simulink model "faultdetectsimulink2"  (R2024b)
settings: Solver=VariableStepAuto  StartTime=0.0  StopTime=0.05  RelTol=1e-3
undefined symbols (not defined in the file or in its folder): D1, Delta
libraries: spsCurrentMeasurementLib x4, spsDistributedParametersLineLib x2, spsThreePhaseVIMeasurementLib x2, spsThreePhaseParallelRLCLoadLib x1, spsThreePhaseTransformerTwoWindingsLib x1, spsThreePhaseFaultLib x1, spsThreePhaseSourceLib x1, sps_lib x1

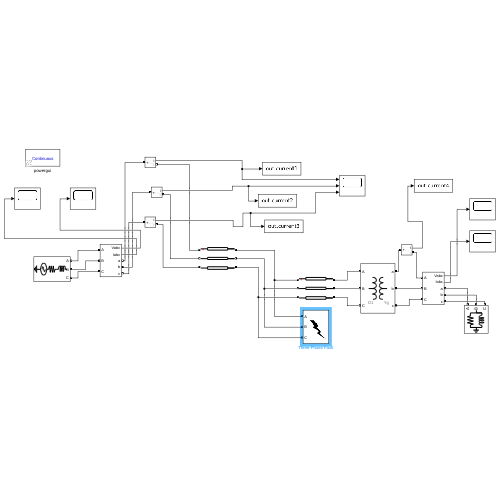
[thumbnail: Simulink's stored preview of the top-level diagram]
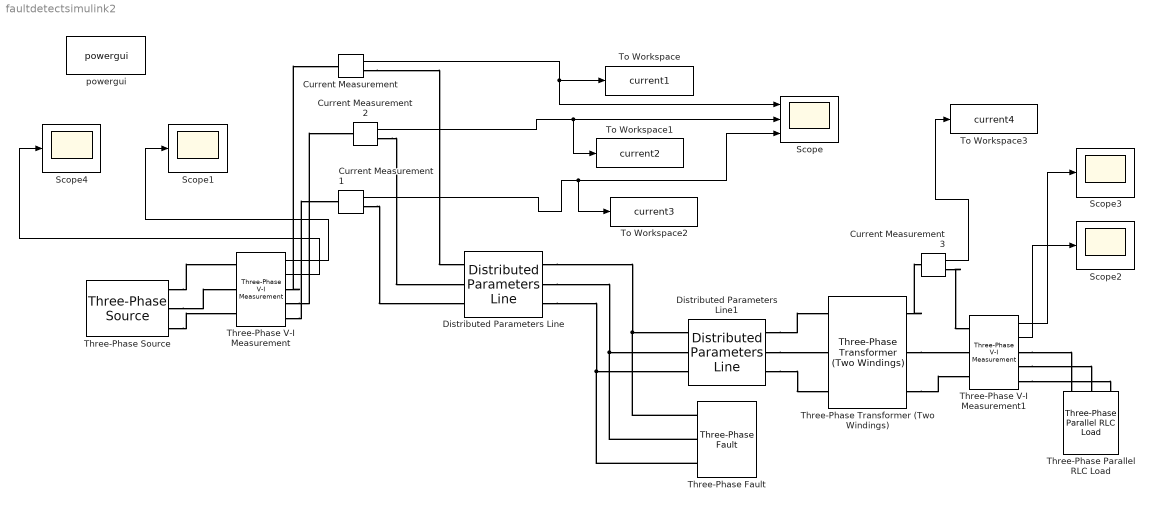
== system faultdetectsimulink2 ==
  Current Measurement{,1..3} (4 alike) : spsCurrentMeasurementLib/Current Measurement  PhasorSimulation=off  OutputType=Complex  PSBequivalent=0
  Distributed Parameters Line : spsDistributedParametersLineLib/Distributed Parameters Line  Phases=3  Length=50  Frequency=50  Resistance=[0.01273 0.3864]  Inductance="[0.9337e-3  4.1264e-3]"  Capacitance=[12.74e-9 7.751e-9]  x1=[3.31061068631267e-12 10912.2714652034 10912.2714652034;314.159265358979 314.159265358979 314.159265358979;-0.367134720613786 0.462312277142197 -1.1084840496527]  x2=[2.03369197834017e-12 10685.5908410511 10685.5908410511;314.159265358979 314.159265358979 314.159265358979;2.58910998298031 0.439349659693703 -1.13144666710119]  x3=[7.88847070447316e-14 26.7116749403581 26.7116749403585;314.159265358979 314.159265358979 314.159265358979;1.48196126518622 1.00491715671543 -0.565879170079457]  x4=[8.43670802456055e-14 59.1805317893528 59.1805317893527;314.159265358979 314.159265358979 314.159265358979;-1.58684353979965 0.173480669902326 -1.39731565689257]  x5=0.000282770783497871  V1=[3.311e-12 1.091e+04 1.091e+04;314.2 314.2 314.2;-0.3671 0.4623 -1.108]  V2=[2.034e-12 1.069e+04 1.069e+04;314.2 314.2 314.2;2.589 0.4393 -1.131]  I1=[7.888e-14 26.71 26.71;314.2 314.2 314.2;1.482 1.005 -0.5659]  I2=[8.437e-14 59.18 59.18;314.2 314.2 314.2;-1.587 0.1735 -1.397]  nHarmo=1  Measurements=None  Decoupling=off  VsMag0=0  VrMag0=0  VsAngle0=0  VrAngle0=0  IsMag0=0  IrMag0=0  IsAngle0=0  IrAngle0=0
      settings: LibrarySourceBlock=sps_lib/Power Grid Elements/Distributed Parameters Line
  Distributed Parameters Line1 : spsDistributedParametersLineLib/Distributed Parameters Line  Phases=3  Length=50  Frequency=50  Resistance=[0.01273 0.3864]  Inductance="[0.9337e-3  4.1264e-3]"  Capacitance=[12.74e-9 7.751e-9]  x1=[2.03369197834017e-12 10685.5908410511 10685.5908410511;314.159265358979 314.159265358979 314.159265358979;2.58910998298031 0.439349659693703 -1.13144666710119]  x2=[1.03798012883211e-11 10433.4111825919 10433.4111825918;314.159265358979 314.159265358979 314.159265358979;-2.16247459933143 0.415478379478156 -1.15531794731674]  x3=[2.26197302864717e-13 26.7063441276431 26.7063441276433;314.159265358979 314.159265358979 314.159265358979;3.02950596917066 1.06083330674248 -0.509963020052391]  x4=[1.49037955982956e-13 59.1198595873729 59.1198595873732;314.159265358979 314.159265358979 314.159265358979;0.100486855906676 0.119677432982979 -1.45111889381193]  x5=0.000282770783497871  V1=[2.034e-12 1.069e+04 1.069e+04;314.2 314.2 314.2;2.589 0.4393 -1.131]  V2=[1.038e-11 1.043e+04 1.043e+04;314.2 314.2 314.2;-2.162 0.4155 -1.155]  I1=[2.262e-13 26.71 26.71;314.2 314.2 314.2;3.03 1.061 -0.51]  I2=[1.49e-13 59.12 59.12;314.2 314.2 314.2;0.1005 0.1197 -1.451]  nHarmo=1  Measurements=None  Decoupling=off  VsMag0=0  VrMag0=0  VsAngle0=0  VrAngle0=0  IsMag0=0  IrMag0=0  IsAngle0=0  IrAngle0=0
      settings: LibrarySourceBlock=sps_lib/Power Grid Elements/Distributed Parameters Line
  Scope : Scope  NumInputPorts=3
  Scope{1..4} (4 alike) : Scope
  Three-Phase Parallel RLC Load : spsThreePhaseParallelRLCLoadLib/Three-Phase Parallel RLC Load  LConnTagsString=A|B|C  Configuration=Y (grounded)  NominalVoltage=400  Vabc=[1e3 1e3 1e3]  Vabcp=[1e3 1e3 1e3]  NominalFrequency=50  UnbalancedPower=off  ActivePower=10e3  InductivePower=100  CapacitivePower=0  Pabc=[10e3 9e3 11e3]  QLabc=[100 90 110]  QCabc=[100 90 110]  Pabcp=[10e3 9e3 11e3]  QLabcp=[100 90 110]  QCabcp=[100 90 110]  Measurements=None  LoadType=constant Z
  Three-Phase Transformer (Two Windings) : spsThreePhaseTransformerTwoWindingsLib/Three-Phase Transformer (Two Windings)  Winding1Connection=Delta (D1)  Winding2Connection=Yg  CoreType=Three single-phase transformers  SetSaturation=off  Hysteresis=off  DataFile='hysteresis'  SetInitialFlux=off  Measurements=None  UNITS=pu  NominalPower=[ 100e6 , 50 ]  Winding1=[ 11e3 , 0.002 , 0.08 ]  Winding2=[ 0.4e3 , 0.002 , 0.08 ]  Rm=500  Lm=500  L0=0.5  Saturation=[ 0,0 ; 0.0024,1.2 ; 1.0,1.52 ]  InitialFluxes=[ 0.8 , -0.8 , 0.7 ]  BreakLoop=off  DiscreteSolver=Trapezoidal iterative  DataType=off  TransfoNumber=1
  Three-Phase V-I Measurement : spsThreePhaseVIMeasurementLib/Three-Phase V-I Measurement  VoltageMeasurement=phase-to-ground  SetLabelV=off  LabelV=Vabc  Vpu=off  VpuLL=off  CurrentMeasurement=yes  SetLabelI=off  LabelI=Iabc  Ipu=off  Pbase=100e6  Vbase=500e3  OutputType=Complex  PhasorSimulation=off  PSBequivalent=0
  Three-Phase V-I Measurement1 : spsThreePhaseVIMeasurementLib/Three-Phase V-I Measurement  VoltageMeasurement=phase-to-ground  SetLabelV=off  LabelV=Vabc  Vpu=off  VpuLL=off  CurrentMeasurement=yes  SetLabelI=off  LabelI=Iabc  Ipu=off  Pbase=100e6  Vbase=500e3  OutputType=Complex  PhasorSimulation=off  PSBequivalent=0
  Three-Phase Fault : spsThreePhaseFaultLib/Three-Phase Fault  InitialStates=0  FaultA=off  FaultB=off  FaultC=off  GroundFault=off  SwitchTimes="[1/60  5/60]"  External=off  SwitchStatus=NaN  FaultResistance=0.01  GroundResistance=0.05  SnubberResistance=1e6  SnubberCapacitance=inf  Measurements=None
  Three-Phase Source : spsThreePhaseSourceLib/Three-Phase Source  InternalConnection=Yg  VoltagePhases=off  Voltage=11e3  PhaseAngle=0  Voltage_phases=[25e3 25e3 25e3]/sqrt(3)  PhaseAngles_phases=[0 -120 +120]  Frequency=50  NonIdealSource=on  SpecifyImpedance=off  Resistance=0.8929  Inductance=16.58e-3  ShortCircuitLevel=100e6  BaseVoltage=11e3  XRratio=7  BusType=swing  Pref=10e3  Qref=0  Prefabc=[10e3, 10e3, 10e3]  Qrefabc=[0, 0, 0]  Qmin=-inf  Qmax=inf
  To Workspace : ToWorkspace  VariableName=current1  SaveFormat=Structure With Time  SampleTime=-1
  To Workspace1 : ToWorkspace  VariableName=current2  SaveFormat=Structure With Time  SampleTime=-1
  To Workspace2 : ToWorkspace  VariableName=current3  SaveFormat=Structure With Time  SampleTime=-1
  To Workspace3 : ToWorkspace  VariableName=current4  SaveFormat=Structure With Time  SampleTime=-1
  powergui : sps_lib/powergui  Priority=1  SimulationMode=Continuous  SampleTime=50e-6  frequency=60  Iterations=50  frequencyindice=50  Pbase=100e6  ErrMax=1e-4  UnitsV=kV  UnitsW=MW  buscounter=0  FunctionMessages=off  echomessages=off  EnableUseOfTLC=off  CurrentSourceSwitches=off  DisableSnubberDevices=off  DisableRonSwitches=off  DisableVfSwitches=off  DisplayEquations=off  AutomaticDiscreteSolvers=off  SolverType=Tustin/Backward Euler (TBE)  Interpol=off  ExternalGateDelay=off  methode=off  Ts=100  x0status=blocks  SPID=on  SwTol=0  HookPort=off  NonlinearTolerance=1e-4  nMaxIteration=100  ContinueOnMaxIteration=off  RestoreLinks=warning  ResistiveCurrentMeasurement=off  Frange=[0:2:500]  Ylog=off  Xlog=on  ShowGrid=off  save=off  variable=ZData  structure=0  ZoomFFT=off  StartTime=0.0  cycles=1  DisplayStyle=1  fundamental=60  FreqAxis=off  MaxFrequency=1000  frequencyindicesteady=1  RmsSteady=1  display=off
  wires:
  Current Measurement/1 -> Scope/1, To Workspace/1
  Current Measurement2/1 -> To Workspace1/1, Scope/2
  Current Measurement1/1 -> To Workspace2/1, Scope/3
  Three-Phase V-I Measurement/1 -> Scope1/1
  Three-Phase V-I Measurement1/1 -> Scope3/1
  Three-Phase V-I Measurement1/2 -> Scope2/1
  Three-Phase V-I Measurement/2 -> Scope4/1
  Current Measurement3/1 -> To Workspace3/1
  connections:
  Three-Phase Source/RConn2 -- Three-Phase V-I Measurement/LConn2
  Three-Phase V-I Measurement/RConn2 -- Current Measurement2/LConn1
  Current Measurement2/RConn1 -- Distributed Parameters Line/LConn2
  Distributed Parameters Line/RConn1 -- Three-Phase Fault/LConn1 -- Distributed Parameters Line1/LConn1
  Distributed Parameters Line/RConn2 -- Three-Phase Fault/LConn2 -- Distributed Parameters Line1/LConn2
  Distributed Parameters Line/RConn3 -- Three-Phase Fault/LConn3 -- Distributed Parameters Line1/LConn3
  Distributed Parameters Line1/RConn2 -- Three-Phase Transformer (Two Windings)/LConn2
  Distributed Parameters Line1/RConn3 -- Three-Phase Transformer (Two Windings)/LConn3
  Three-Phase Transformer (Two Windings)/RConn2 -- Three-Phase V-I Measurement1/LConn2
  Three-Phase Transformer (Two Windings)/RConn3 -- Three-Phase V-I Measurement1/LConn3
  Three-Phase V-I Measurement1/RConn1 -- Three-Phase Parallel RLC Load/LConn1
  Three-Phase V-I Measurement1/RConn2 -- Three-Phase Parallel RLC Load/LConn2
  Three-Phase V-I Measurement1/RConn3 -- Three-Phase Parallel RLC Load/LConn3
  Current Measurement/RConn1 -- Distributed Parameters Line/LConn1
  Three-Phase V-I Measurement/RConn1 -- Current Measurement/LConn1
  Three-Phase Source/RConn3 -- Three-Phase V-I Measurement/LConn3
  Three-Phase V-I Measurement/RConn3 -- Current Measurement1/LConn1
  Current Measurement1/RConn1 -- Distributed Parameters Line/LConn3
  Three-Phase Source/RConn1 -- Three-Phase V-I Measurement/LConn1
  Distributed Parameters Line1/RConn1 -- Three-Phase Transformer (Two Windings)/LConn1
  Three-Phase Transformer (Two Windings)/RConn1 -- Current Measurement3/LConn1
  Current Measurement3/RConn1 -- Three-Phase V-I Measurement1/LConn1
